simulink model "Ljap_Reg_S_2"  (R2023b)
settings: Solver=ode45  StartTime=0.0  StopTime=15  RelTol=1e-5  AbsTol=1e-5  EnableMultiTasking=on
model workspace (MAT data in the model file):
  Am = [-1.66666666667  0  0; 0  0  1; 0  -0.444444444444  -1.33333333333]
  Beta = [50  0  0; 0  50  0; 0  0  50]
  Bm = [1.66666666667  0; 0  0; 0  0.444444444444]
  Delta = [10  0  0; 0  10  0; 0  0  10]
  P = [-30  -16.3265306122  61.2244897959; -16.3265306122  -18.5416666667  -1.125; 61.2244897959  -1.125  -38.34375]
  T1 = 0.6
  T2 = 1.5
  a1 = -0.99
  b1 = -3.44
  c1 = 0.03
  d1 = 2.06
  e1 = -0.37
  v = -0.32
settings Model: Creator=PF  LastModifiedBy=ivanz
settings SolverCC: AutoScaleAbsTol=off  AlgebraicLoopSolver=TrustRegion
settings DataIOCC: LimitDataPoints=on  SaveFormat=Array  SignalLoggingSaveFormat=ModelDataLogs  ReturnWorkspaceOutputs=off  SignalLoggingName=sigsOut
settings OptimizationCC: InitFltsAndDblsToZero=on  LifeSpan=inf
settings DebuggingCC: SaveWithParameterizedLinksMsg=none  UnderspecifiedInitializationDetection=Classic  MergeDetectMultiDrivingBlocksExec=none  SignalResolutionControl=TryResolveAllWithWarning  MultiTaskDSMMsg=warning  MultiTaskCondExecSysMsg=none  FcnCallInpInsideContextMsg=warning  UnconnectedInputMsg=warning  UnconnectedOutputMsg=warning  UnconnectedLineMsg=warning  SFUnexpectedBacktrackingDiag=warning  SFNoUnconditionalDefaultTransitionDiag=warning  SFExecutionAtInitializationDiag=none  ArithmeticOperatorsInVariantConditions=warning
settings HardwareCC: ProdBitPerPointer=32  ProdBitPerSizeT=32  ProdBitPerPtrDiffT=32  ProdLargestAtomicFloat=None  ProdIntDivRoundTo=Undefined  ProdEndianess=Unspecified  ProdWordSize=32  ProdHWDeviceType=32-bit Generic  TargetUnknown=on
settings ModelReferenceCC: EnableRefExpFcnMdlSchedulingChecks=on  PropagateSignalLabelsOutOfModel=off
settings RTWCC: DLArmComputeVersion=19.05
settings CodeAppCC: StateflowObjectComments=on
settings GRTTargetCC: TargetFcnLib=ansi_tfl_tmw.mat  TargetLangStandard=C89/C90 (ANSI)  CombineOutputUpdateFcns=off  GRTInterface=on
settings ConfigComp: CovMetricSettings=dw  CovSaveCumulativeToWorkspaceVar=on  CovSaveSingleToWorkspaceVar=on

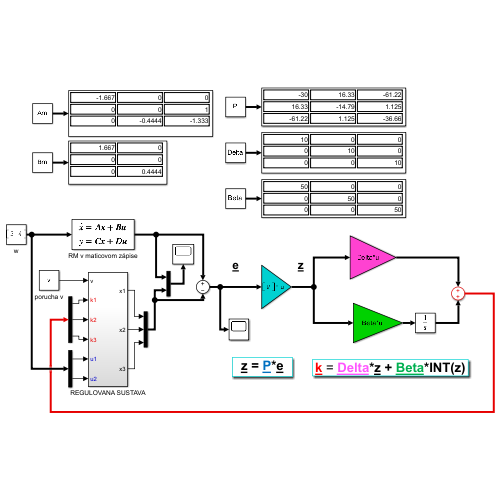
[thumbnail: Simulink's stored preview of the top-level diagram]
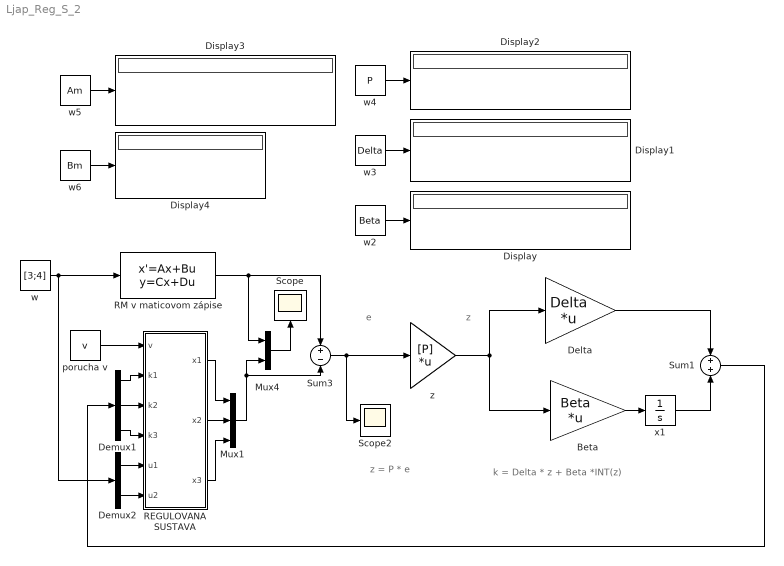
== system Ljap_Reg_S_2 ==
  note: z
  note: z = P * e
  note: k = Delta * z + Beta *INT(z)
  note: e
  Beta : Gain  Gain=Beta  Multiplication=Matrix(K*u)  SaturateOnIntegerOverflow=on  OutDataTypeStr=Inherit: Same as input  ParamDataTypeStr=Inherit: Same as input
  Delta : Gain  Gain=Delta  Multiplication=Matrix(K*u)  SaturateOnIntegerOverflow=on  OutDataTypeStr=Inherit: Same as input  ParamDataTypeStr=Inherit: Same as input
  Demux1 : Demux  Outputs=3
  Demux2 : Demux  Outputs=2
  Display{,1..4} (5 alike) : Display
  Mux1 : Mux  Inputs=3
  Mux4 : Mux  Inputs=2
  REGULOVANA SUSTAVA : Subsystem
  RM v maticovom zápise : StateSpace  A=[-1/T1 0 0; 0 0 1; 0 -1/T2^2 -2/T2]  B=[1/T1 0; 0 0; 0 1/T2^2]  C=[1 0 0;0 1 0; 0 0 1]  D=[0 0;0 0;0 0]  InitialCondition=0
  Scope : Scope
  Scope2 : Scope
  Sum1 : Sum  SaturateOnIntegerOverflow=on
  Sum3 : Sum  Inputs=+-  SaturateOnIntegerOverflow=on
  porucha v : Constant  Value=v
  w : Constant  Value=[3;4]
  w2 : Constant  Value=Beta
  w3 : Constant  Value=Delta
  w4 : Constant  Value=P
  w5 : Constant  Value=Am
  w6 : Constant  Value=Bm
  x1 : Integrator
  z : Gain  Gain=[P]  Multiplication=Matrix(K*u)  SaturateOnIntegerOverflow=on  OutDataTypeStr=Inherit: Same as input  ParamDataTypeStr=Inherit: Same as input
  wires:
  RM v maticovom zápise/1 -> Mux4/1, Sum3/1
  w/1 -> RM v maticovom zápise/1, Demux2/1
  porucha v/1 -> REGULOVANA SUSTAVA/1(v)
  Beta/1 -> x1/1
  x1/1 -> Sum1/2
  Delta/1 -> Sum1/1
  z/1 -> Delta/1, Beta/1
  Sum3/1 -> Scope2/1, z/1
  w2/1 -> Display/1
  w3/1 -> Display1/1
  w4/1 -> Display2/1
  w5/1 -> Display3/1
  w6/1 -> Display4/1
  Sum1/1 -> Demux1/1
  Mux1/1 -> Mux4/2, Sum3/2
  Mux4/1 -> Scope/1
  Demux1/2 -> REGULOVANA SUSTAVA/3(k2)
  Demux1/1 -> REGULOVANA SUSTAVA/2(k1)
  Demux1/3 -> REGULOVANA SUSTAVA/4(k3)
  REGULOVANA SUSTAVA/1(x1) -> Mux1/1
  REGULOVANA SUSTAVA/2(x2) -> Mux1/2
  REGULOVANA SUSTAVA/3(x3) -> Mux1/3
  Demux2/1 -> REGULOVANA SUSTAVA/5(u1)
  Demux2/2 -> REGULOVANA SUSTAVA/6(u2)

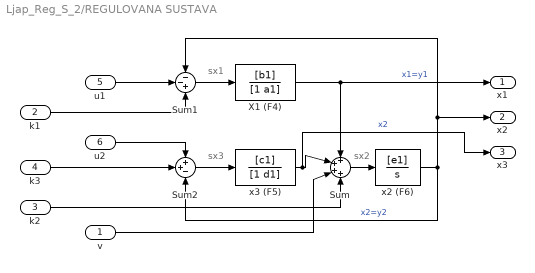
== system Ljap_Reg_S_2/REGULOVANA SUSTAVA ==
  note: sx1
  note: sx3
  note: sx2
  v : Inport
  k1 : Inport  Port=2
  k2 : Inport  Port=3
  k3 : Inport  Port=4
  u1 : Inport  Port=5
  u2 : Inport  Port=6
  Sum : Sum  Inputs=++++
  Sum1 : Sum  Inputs=--+
  Sum2 : Sum  Inputs=++-
  X1 (F4) : TransferFcn  Numerator=[b1]  Denominator=[1 a1]
  x2 (F6) : TransferFcn  Numerator=[e1]  Denominator=[1 0]
  x3 (F5) : TransferFcn  Numerator=[c1]  Denominator=[1 d1]
  x1 : Outport
  x2 : Outport  Port=2
  x3 : Outport  Port=3
  wires:
  x2 (F6)/1 -> x2/1, Sum1/1, Sum2/3  "x2=y2"
  Sum1/1 -> X1 (F4)/1
  u1/1 -> Sum1/2
  v/1 -> Sum/3
  k1/1 -> Sum1/3
  Sum2/1 -> x3 (F5)/1
  Sum/1 -> x2 (F6)/1
  x3 (F5)/1 -> x3/1, Sum/2  "x2"
  X1 (F4)/1 -> x1/1, Sum/1  "x1=y1"
  u2/1 -> Sum2/1
  k3/1 -> Sum2/2
  k2/1 -> Sum/4
